simulink model "DriveTrainModel2"  (R2025a)
settings: Solver=VariableStepAuto  StartTime=0.0  StopTime=10.0  FixedStep=0.01  RelTol=1e-3
undefined symbols (not defined in the file): L, R
settings Model: DataDictionary=Constants.sldd  Creator=levirogalla  LastModifiedBy=levirogalla

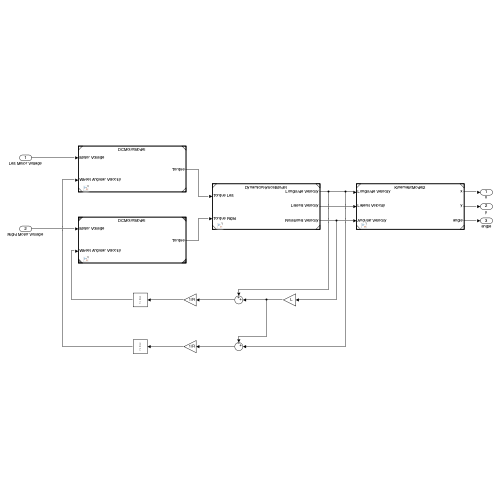
[thumbnail: Simulink's stored preview of the top-level diagram]
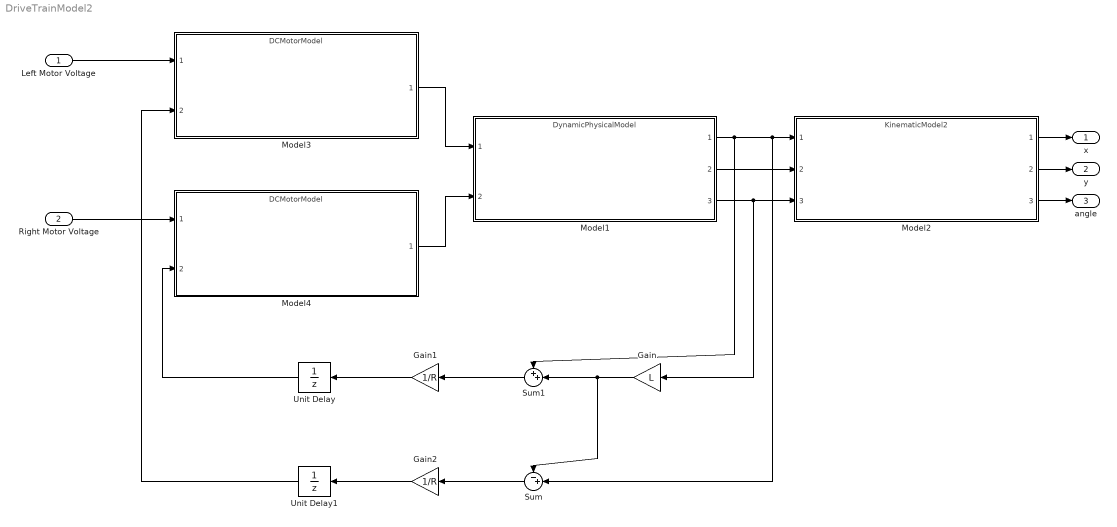
== system DriveTrainModel2 ==
  Left Motor Voltage : Inport
  Right Motor Voltage : Inport  Port=2
  Gain : Gain  Gain=L
  Gain1 : Gain  Gain=1/R
  Gain2 : Gain  Gain=1/R
  Model1 : ModelReference  ModelNameDialog=DynamicPhysicalModel.slx  SimulationMode=Normal  ModelReferenceVersion=3.1
  Model2 : ModelReference  ModelNameDialog=KinematicModel2.slx  SimulationMode=Normal  ModelReferenceVersion=3.1
  Model3 : ModelReference  ModelNameDialog=DCMotorModel.slx  SimulationMode=Normal  ModelReferenceVersion=3.1
  Model4 : ModelReference  ModelNameDialog=DCMotorModel.slx  SimulationMode=Normal  ModelReferenceVersion=3.1
  Sum : Sum  Inputs=-+|
  Sum1 : Sum  Inputs=++|
  Unit Delay : UnitDelay  SampleTime=-1  HasFrameUpgradeWarning=on
  Unit Delay1 : UnitDelay  SampleTime=-1  HasFrameUpgradeWarning=on
  x : Outport
  y : Outport  Port=2
  angle : Outport  Port=3
  wires:
  Model1/3 -> Gain/1, Model2/3
  Sum/1 -> Gain2/1
  Gain/1 -> Sum/1, Sum1/2
  Model1/1 -> Sum1/1, Sum/2, Model2/1
  Model3/1 -> Model1/1
  Sum1/1 -> Gain1/1
  Model1/2 -> Model2/2
  Model4/1 -> Model1/2
  Left Motor Voltage/1 -> Model3/1
  Right Motor Voltage/1 -> Model4/1
  Model2/1 -> x/1
  Model2/2 -> y/1
  Model2/3 -> angle/1
  Gain1/1 -> Unit Delay/1
  Gain2/1 -> Unit Delay1/1
  Unit Delay/1 -> Model4/2
  Unit Delay1/1 -> Model3/2
